simulink model "example7"  (Simulink 7.1)
settings: Solver=ode45  StartTime=0.0  StopTime=1.5  MaxStep=0.01  RelTol=1e-3
model workspace: external: M-Code (data not in the file)
undefined symbols (not defined in the file or in its folder): Fpt, gcontact, npoly, npt, x_init
libraries: simulink x6
settings Model: Creator=roy  LastModifiedBy=roy
settings DataIOCC: LimitDataPoints=off

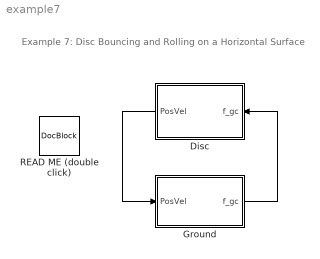
== system example7 ==
  note: Example 7: Disc Bouncing and Rolling
      | on a Horizontal Surface
  Disc : Subsystem  Orientation=left
  Ground : Subsystem
  READ ME (double click) : simulink/Model-Wide Utilities/DocBlock  SystemSampleTime=-1  DocumentType=Text
      content=|
      | This Simulink model shows how to use the ground-contact model, which
      | allows you to simulate the effect of physical contact between a rigid-body
      | system and a compliant ground plane.  In this case, the system consists of
      | a polyhedral approximation to a disc which falls under gravity, hits the
      | ground, bounces a bit, and then rolls with a bit of a wobble until the end
      | of the simulation.  The wobble is deliberate, and is caused by the disc
      | hitting the ground at an angle.
      |
      | This simulation is ready to run: just click on "start" in the simulation
      | menu, and watch the signals appear in the scope window.  To see the
      | resulting motion with showmotion, use the command
      | "showmotion(rollingdisc(16),tout,fbanim(xout))".  The argument 16 tells
      | rollingdisc how many vertices to use in its polygonal approximation to a
      | circle, and it must be the same as the number used in the simulation.  The
      | disc produced by rollingdisc is quite small (just 10cm in diameter), so
      | the motion happens quite quickly, and the whole simulation lasts just 1.5
      | seconds.  So you will probably want to view it in slow motion.  You will
      | also notice that showmotion is using a tracking camera in order to follow
      | the disc as it rolls.
      |
      | Now that you've seen the motion, here are some technical details to
      | explain what is going on.  First, the system model produced by rollingdisc
      | contains a special field called gc, which declares a set of points that
      | can make contact with the ground.  You can take a look by first typing
      | "disc=rollingdisc(16);" and then "disc.gc".  Each point is defined by the
      | body number of the body to which it belongs, and its coordinates expressed
      | in the local coordinate system of that body.  In this particular case,
      | every point is attached to body 6 (the floating base).  The ground-contact
      | model now works as follows:
      |
      | 1. A special function (gcPosVel) calculates a matrix containing the
      |    position and velocity of every point described in the field gc.
      |
      | 2. Another special function (gcontact) calculates the ground-reaction
      |    force acting on each point, as a function of its position and
      |    velocity.
      |
      | 3. A third special function (gcFD, which first appeared in example 5)
      |    converts these forces into the format required by the dynamics
      |    functions in their f_ext argument, and then calls a dynamics function.
      |
      | The end result is that the disc moves in response to gravity and the
      | ground-reaction forces it experiences as it comes into contact with the
      | ground.
      |
      | You can find gcPosVel and gcFD in the subsystem "disc" and gcontact in the
      | subsystem "ground".  You can also find more detailed documentation on how
      | the ground-contact model works in those subsystems.
      |
      | Here are some experiments you can try.  First, open the model explorer
      | (using the "view" menu), and open the model workspace of example7 (in the
      | left-hand pane).  You will now see a small amount of Matlab code (m-code)
      | in the right-hand pane that you can edit directly.  Remember: each time
      | you make a change to this code, you must first press "Apply" and then
      | "Reinitialize from Source" before your changes take effect.  Now try
      | these:
      |
      | 1. Change "npoly" from 16 to 60.  This will give you a much better
      |    approximation to a circular disc.  To view the results with showmotion,
      |    use "showmotion(rollingdisc(60),tout,fbanim(xout))".  You can also try
      |    numbers smaller than 16.
      |
      | 2. Change "npoly" back to 16, and change "ta" from 0.18 to 0.22.  This
      |    parameter is the twist angle (radians) with which the disc hits the
      |    ground.  Increasing it to 0.22 is enough to make the disc fall over.
      |    Observe that the disc slips as it falls.  This is because the ground is
      |    very slippery (its friction coefficient has been set quite low).
  wires:
  Disc/1(PosVel) -> Ground/1(PosVel)
  Ground/1(f_gc) -> Disc/1(f_gc)

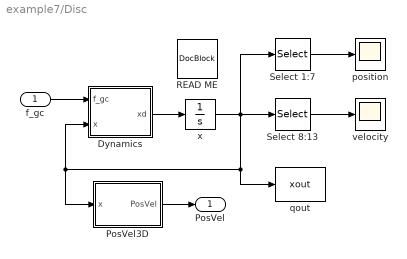
== system example7/Disc ==
  f_gc : Inport  OutDataType=sfix(16)  OutScaling=2^0
  Dynamics : Subsystem
  PosVel3D : Subsystem
  READ ME : simulink/Model-Wide Utilities/DocBlock  SystemSampleTime=-1  DocumentType=Text
      content=|
      | This subsystem builds upon the dynamics calculation in Example 4
      | (free-floating single rigid body).  The two new elements here are: a new
      | argument (f_gc) input to the dynamics calculation, and a new subsystem to
      | calculate the positions and velocities of the ground-contact points.
      |
      | Inside the "Dynamics" subsystem you will find that the floating-base state
      | vector, x, has been combined with the constant npoly and the matrix of
      | ground-contact forces, f_gc.  npoly is required as an argument to
      | rollingdisc.  The reason why it has to be supplied as an input like this
      | is because the executable expression in a "MATLAB Function" block does not
      | have access to the Simulink model's workspace (which is where npoly is
      | defined), so the symbol "npoly" cannot appear directly in this
      | expression.  f_gc is a 6x(npt) matrix, where npt is the number of points
      | defined in the rolling disc model, such that f_gc(:,i) is the spatial
      | force acting on point number i.  The "reshape" block converts it to a
      | column vector such that the first column of f_gc appears in the first six
      | elements, the second column in the next six elements, and so on.  The
      | function gcFD (appearing inside the "MATLAB Function" block) converts this
      | data into the cell-array format required by the f_ext arguments of the
      | dynamics functions, and calls FDfb to calculate the floating-base forward
      | dynamics of the rolling disc.
      |
      | Inside the "PosVel3D" subsystem, you will find the call to gcPosVel.  Once
      | again, npoly is supplied as a constant input, because it is needed as an
      | argument to rollingdisc but cannot appear explicitly in the executable
      | expression in the "MATLAB Function" block.  This function calculates a
      | 6x(npt) matrix such that column i contains the position (first three
      | elements) and velocity (last three elements) of point number i, both
      | expressed in base (body 0) coordinates.
      |
      | This dynamics subsystem can easily be adapted to fixed-base system models,
      | to floating-base models with more than one body, and to system models
      | based on planar arithmetic.  In the case of planar arithmetic, the
      | incoming f_gc is a 3x(npt) matrix whose columns are planar force vectors,
      | and the matrix calculated by gcPosVel is a 4x(npt) matrix containing two
      | 2D vectors in each column.  If vectors of joint position and velocity
      | variables (q and qd) are required instead of or in addition to x, then
      | these must be supplied as inputs to both gcFD and gcPosVel; so you will
      | have to add extra input ports to the blocks "Dynamics" and "PosVel3D".
  Select 1:7 : Selector  InputPortWidth=13  IndexOptions=Index vector (dialog)  Indices=[1 2 3 4 5 6 7]  OutputSizes=1
  Select 8:13 : Selector  InputPortWidth=13  IndexOptions=Index vector (dialog)  Indices=[8 9 10 11 12 13]  OutputSizes=1
  position : Scope
      settings: YMin=-1.05  YMax=1.05
  qout : ToWorkspace  VariableName=xout  SampleTime=-1  SaveFormat=Array
  velocity : Scope
      settings: YMin=-2  YMax=4  SaveName=ScopeData2
  x : Integrator  InitialCondition=x_init
  PosVel : Outport  OutDataType=sfix(16)  OutScaling=2^0
  wires:
  PosVel3D/1(PosVel) -> PosVel/1
  f_gc/1 -> Dynamics/1(f_gc)
  Dynamics/1(xd) -> x/1
  Select 1:7/1 -> position/1
  Select 8:13/1 -> velocity/1
  x/1 -> Select 8:13/1, Select 1:7/1, Dynamics/2(x), PosVel3D/1(x), qout/1

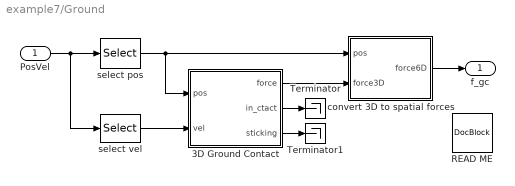
== system example7/Ground ==
  PosVel : Inport  OutDataType=sfix(16)  OutScaling=2^0
  3D Ground Contact : Subsystem  mask(3D Nonlinear Ground Contact with Friction){K=1e6, D=2000, mu=0.1, np=npt}
      mask prompts: K "Stiffness (K)"; D "Damping (D)"; mu "Coefficient of Friction (mu)"; np "Number of Contact Points"
      mask help:
      | Given two 3xnp arrays containing contact-point positions and
      | velocities, calculate the 3xnp array of ground-reaction forces
      | acting on those points. Also calculate 1xnp boolean vectors
      | in_ctact (true if normal force >0) and sticking (true if inside
      | or on boundary of friction cone).  Zero-crossing detection is
      | enabled at both make/break contact and stick/slip transitions.
  READ ME : simulink/Model-Wide Utilities/DocBlock  SystemSampleTime=-1  DocumentType=Text
      content=|
      | This subsystem implements the Simulink ground-contact model in 3D.  The
      | input is a 6x(npt) matrix such that column i contains the 3D position (top
      | 3 elements) and linear velocity (bottom 3 elements) of ground-contact
      | point number i (i.e., the i^th point defined in the "gc" field of the
      | system model data structure).  The output is a 6x(npt) matrix such that
      | column i is the spatial force acting on point number i.  All quantities
      | are expressed in base (body 0) coordinates.
      |
      | The first thing that happens is that the input matrix is split into
      | separate position and velocity matrices.  Both are then sent to the "3D
      | Ground Contact" subsystem, which calculates the force acting on each
      | point.  The "force" output is a 3x(npt) matrix of linear forces, which is
      | converted to a matrix of spatial forces by the final block in the
      | subsystem.  The other two outputs are 1x(npt) arrays of Boolean variables
      | such that in_ctact(i) is true if point i is in contact with the ground
      | (meaning that it is experiencing a nonzero force) and sticking(i) is true
      | if point i is sticking (due to friction) to the ground.
      |
      | The subsystem "3D Ground Contact" is a masked subsystem.  If you
      | double-click on this block then you will get a dialog window displaying
      | the following parameters: Stiffness (K), Damping (D), coefficient of
      | friction (mu), and Number of Contact Points.  The first three must be
      | strictly-positive scalars, and the fourth must equal the number of points
      | defined in the "gc" field of the system model data structure.  The current
      | settings of K, D and mu correspond to a soft, very slippery plastic
      | surface.  Increasing K will make it harder, and increasing the ratio K/D
      | will make it bouncier, but be aware that both increase the stiffness of
      | the differential equations that Simulink is solving, meaning that Simulink
      | will be forced to take smaller steps.  A typical value of mu for a safe
      | (non-slip) floor is 0.5.
      |
      | To see how this subsystem is implemented, you will have to look under the
      | mask.  You can do that by right-clicking on the block and selecting the
      | menu option "Look Under Mask".  There, you will find that this block is
      | based on the function gcontact, and you will also find a bit more
      | documentation.
  Terminator : Terminator
  Terminator1 : Terminator
  convert 3D to spatial forces : Subsystem
  select pos : Selector  NumberOfDimensions=2  InputPortWidth=3  IndexOptions=Index vector (dialog),Select all  Indices=[1 2 3],1  OutputSizes=1,1
  select vel : Selector  NumberOfDimensions=2  InputPortWidth=3  IndexOptions=Index vector (dialog),Select all  Indices=[4 5 6],1  OutputSizes=1,1
  f_gc : Outport  OutDataType=sfix(16)  OutScaling=2^0
  wires:
  PosVel/1 -> select pos/1, select vel/1
  select pos/1 -> convert 3D to spatial forces/1(pos), 3D Ground Contact/1(pos)
  convert 3D to spatial forces/1(force6D) -> f_gc/1
  select vel/1 -> 3D Ground Contact/2(vel)
  3D Ground Contact/1(force) -> convert 3D to spatial forces/2(force3D)
  3D Ground Contact/2(in_ctact) -> Terminator/1
  3D Ground Contact/3(sticking) -> Terminator1/1

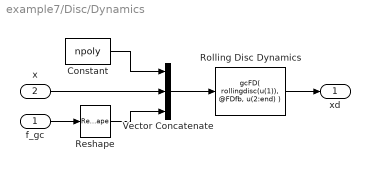
== system example7/Disc/Dynamics ==
  f_gc : Inport  OutDataType=sfix(16)  OutScaling=2^0
  x : Inport  Port=2  OutDataType=sfix(16)  OutScaling=2^0
  Constant : Constant  Value=npoly  OutDataType=sfix(16)  OutScaling=2^0
  Reshape : Reshape  OutputDimensionality=Column vector (2-D)
  Rolling Disc Dynamics : MATLABFcn  MATLABFcn=gcFD( rollingdisc(u(1)), @FDfb, u(2:end) )  OutputDimensions=[13 1]  OutputSignalType=real  Output1D=off
  Vector Concatenate : Concatenate  NumInputs=3  Mode=Vector
  xd : Outport  OutDataType=sfix(16)  OutScaling=2^0
  wires:
  f_gc/1 -> Reshape/1
  Vector Concatenate/1 -> Rolling Disc Dynamics/1
  Rolling Disc Dynamics/1 -> xd/1
  Reshape/1 -> Vector Concatenate/3
  x/1 -> Vector Concatenate/2
  Constant/1 -> Vector Concatenate/1

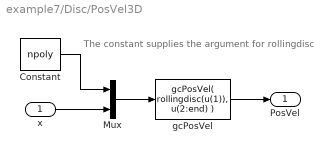
== system example7/Disc/PosVel3D ==
  note: The constant supplies the
      | argument for rollingdisc
  x : Inport  OutDataType=sfix(16)  OutScaling=2^0
  Constant : Constant  Value=npoly  OutDataType=sfix(16)  OutScaling=2^0
  Mux : Mux  Inputs=2
  gcPosVel : MATLABFcn  MATLABFcn=gcPosVel( rollingdisc(u(1)), u(2:end) )  OutputDimensions=[6 npt]  OutputSignalType=real  Output1D=off
  PosVel : Outport  OutDataType=sfix(16)  OutScaling=2^0
  wires:
  gcPosVel/1 -> PosVel/1
  Mux/1 -> gcPosVel/1
  x/1 -> Mux/2
  Constant/1 -> Mux/1

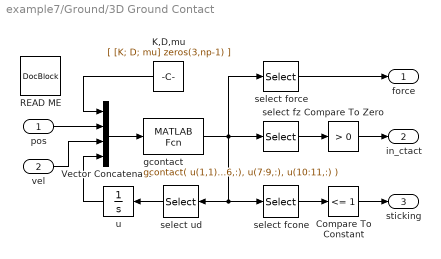
== system example7/Ground/3D Ground Contact ==
  pos : Inport  OutDataType=sfix(16)  OutScaling=2^0
  vel : Inport  Port=2  OutDataType=sfix(16)  OutScaling=2^0
  Compare To Constant : simulink/Logic and Bit Operations/Compare To Constant  SystemSampleTime=-1  relop=<=  const=1  LogicOutDataTypeMode=boolean
  Compare To Zero : simulink/Logic and Bit Operations/Compare To Zero  SystemSampleTime=-1  relop=>  LogicOutDataTypeMode=boolean
  K,D,mu : Constant  Orientation=left  Value=[ [K; D; mu] zeros(3,np-1) ]  VectorParams1D=off  OutDataType=sfix(16)  OutScaling=2^0
  READ ME : simulink/Model-Wide Utilities/DocBlock  SystemSampleTime=-1  DocumentType=Text
      content=|
      | The constant block supplies the parameters K, D and mu to the function
      | gcontact.  This is necessary because K, D and mu are defined in the
      | workspace of this particular masked subsystem, but the executable
      | expression in the "MATLAB Function" block does not have access to this
      | workspace, so the symbols K, D and mu cannot appear directly in the
      | executable expression.
      |
      | The ">0" block and the "<=1" block both have zero-crossing enabled.  The
      | former detects transitions between contact and non-contact, whereas the
      | latter detects transitions between sticking (due to friction) and
      | slipping.  A point can be sticking only if it is also in contact.  A
      | zero-crossing event occurs whenever any one point makes a transition.
      |
      | The state variable, u, is a 2x(np) matrix containing the horizontal
      | component of the local ground deformation for each point.  This quantity
      | is used to calculate the tangential (i.e., frictional) component of the
      | ground reaction force.
      |
      | When a point loses contact, its associated state variable, u(:,i), decays
      | to zero with a time constant of D/K.  If this ratio is small then the
      | corresponding differential equation is fast, and it is necessary to use
      | small integration time steps.  For example, if K=1e6 and D=2000 then
      | D/K=0.002 and u(:,i) decays in proportion to exp(-500t).  Increasing K
      | makes the surface stiffer, and decreasing D/K makes it bouncier, but the
      | latter also makes the post-contact recovery faster.  The degree of
      | bounciness depends on the mass of the impacting body: a heavier body will
      | bounce more.
      |
      | To adapt this subsystem to work in 2D, the only things that change are the
      | row dimensions of various matrices.  You will have to alter the row
      | selections in the executable expression in the "MATLAB Function" block,
      | and also the dimensions of its output matrix, and you will have to change
      | the row selections in the various "select" blocks.
      |
      | For more information, see "The Simulink Ground Contact Model" in the
      | spatial_v2 documentation directory.
  Vector Concatenate : Concatenate  NumInputs=4  Mode=Multidimensional array
  gcontact : MATLABFcn  MATLABFcn=gcontact( u(1,1), u(2,1), u(3,1), u(4:6,:), u(7:9,:), u(10:11,:) )  OutputDimensions=[6 np]  OutputSignalType=real  Output1D=off
  select fcone : Selector  NumberOfDimensions=2  InputPortWidth=3  IndexOptions=Index vector (dialog),Select all  Indices=[6],1  OutputSizes=1,1
  select force : Selector  NumberOfDimensions=2  InputPortWidth=3  IndexOptions=Index vector (dialog),Select all  Indices=[1 2 3],1  OutputSizes=1,1
  select fz : Selector  NumberOfDimensions=2  InputPortWidth=3  IndexOptions=Index vector (dialog),Select all  Indices=[3],1  OutputSizes=1,1
  select ud : Selector  Orientation=left  NumberOfDimensions=2  InputPortWidth=3  IndexOptions=Index vector (dialog),Select all  Indices=[4 5],1  OutputSizes=1,1
  u : Integrator  Orientation=left
  force : Outport  OutDataType=sfix(16)  OutScaling=2^0
  in_ctact : Outport  Port=2  OutDataType=sfix(16)  OutScaling=2^0
  sticking : Outport  Port=3  OutDataType=sfix(16)  OutScaling=2^0
  wires:
  Vector Concatenate/1 -> gcontact/1
  select ud/1 -> u/1
  gcontact/1 -> select force/1, select fz/1, select ud/1, select fcone/1
  select force/1 -> force/1
  select fz/1 -> Compare To Zero/1
  Compare To Zero/1 -> in_ctact/1
  select fcone/1 -> Compare To Constant/1
  Compare To Constant/1 -> sticking/1
  u/1 -> Vector Concatenate/4
  vel/1 -> Vector Concatenate/3
  pos/1 -> Vector Concatenate/2
  K,D,mu/1 -> Vector Concatenate/1

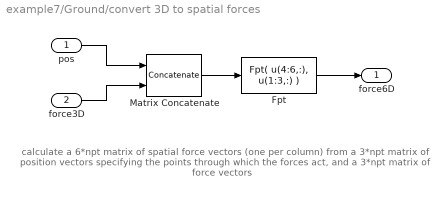
== system example7/Ground/convert 3D to spatial forces ==
  note: calculate a 6*npt matrix of spatial force vectors (one per column)
      | from a 3*npt matrix of position vectors specifying the points
      | through which the forces act, and a 3*npt matrix of force vectors
  pos : Inport  OutDataType=sfix(16)  OutScaling=2^0
  force3D : Inport  Port=2  OutDataType=sfix(16)  OutScaling=2^0
  Fpt : MATLABFcn  MATLABFcn=Fpt( u(4:6,:), u(1:3,:) )  OutputSignalType=real  Output1D=off
  Matrix Concatenate : Concatenate  Mode=Multidimensional array
  force6D : Outport  OutDataType=sfix(16)  OutScaling=2^0
  wires:
  force3D/1 -> Matrix Concatenate/2
  pos/1 -> Matrix Concatenate/1
  Matrix Concatenate/1 -> Fpt/1
  Fpt/1 -> force6D/1
